simulink model "AE426SIMULINK8_OLD_viewerV2"  (R2024b)
settings: Solver=ode4  StartTime=0  StopTime=simlength  FixedStep=dt  RelTol=1e-3
InitFcn:
  | clear
  | clf
  | close all
  | wrlFilePath = fullfile(pwd, 'SpacecraftEarth.wrl');
  | myworld = vrworld(wrlFilePath);
  | open(myworld);
  | set(0,'Units','pixels');
  | 
  | screenSize = get(0, 'ScreenSize');
  | screenWidth = screenSize(3);
  | screenHeight = screenSize(4);
  | figWidth = screenWidth / 3;
  | figHeight = screenHeight / 2;
  | 
  | positions = [
  |      screenHeight - figHeight, 0, figWidth, figHeight; % Top-left
  |      figWidth, screenHeight - figHeight, figWidth, figHeight; % Top-right
  |      2*figWidth, screenHeight - figHeight, figWidth, figHeight; % Bottom-left
  | ];
  | 
  | fig1 = vrfigure(myworld,positions(1, :));
  | set(fig1,'Viewpoint','WorldView');
  | 
  | fig2 = vrfigure(myworld,positions(2, :));
  | set(fig2,'Viewpoint','NadirView');
  | 
  | fig3 = vrfigure(myworld,positions(3, :));
  | set(fig3,'Viewpoint','TargetView');
  | 
  | vrsetpref DefaultFigurePlaneClipMethod bvolume
  | 
  | % CONFIGURATION GOEMETRY MODELLING
  | 
  | fuse_dia = 0.3; % m
  | fuse_L = 0.9; %m
  | braket_space = 0.05; % m
  | num_ab = 3;
  | ab_span = 0.9; % m
  | ab_chord = 0.6844; % m
  | sys_CG = [-.01641,.06324,-.40481]; % m; respect to top of fuselage
  | 
  | CYLc = [0,0,.45] + sys_CG;
  | ab_cd = 2.2;
  | cyl_cd = 0.8;
  | 
  | mu = 3.986004e5;
  | dt = 0.01;
  | % ypr0 = [pi/4,pi/6,-pi/6];
  | % q1 = sin(ypr0(3)/2)*cos(ypr0(2)/2)*cos(ypr0(1)/2)-cos(ypr0(3)/2)*sin(ypr0(2)/2)*sin(ypr0(1)/2);
  | % q2 = sin(ypr0(3)/2)*cos(ypr0(2)/2)*sin(ypr0(1)/2)+cos(ypr0(3)/2)*sin(ypr0(2)/2)*cos(ypr0(1)/2);
  | % q3 = cos(ypr0(3)/2)*cos(ypr0(2)/2)*sin(ypr0(1)/2)-sin(ypr0(3)/2)*sin(ypr0(2)/2)*cos(ypr0(1)/2);
  | % q4 = cos(ypr0(3)/2)*cos(ypr0(2)/2)*cos(ypr0(1)/2)+sin(ypr0(3)/2)*sin(ypr0(2)/2)*sin(ypr0(1)/2);
  | % q0 = [q1;q2;q3;q4];
  | q0 = [0;0;0;1];
  | w0 = [0.000;0.000;0.000];
  | H0 = [0;0;0];
  | lat = [34.6178 34.9438 34.3658].*pi./180;
  | long = [-112.4503 -111.7529 -111.4481].*pi./180;
  | longlat = [long;lat]';
  | 
  | ... (+72 lines)
StopFcn:
  | data = get(out,"YPR");
  | data_e1 = get(out,"TargetYPR");
  | t = data.time - 51744.4;
  | 
  | y = data.Data(:,1);
  | p = data.Data(:,2);
  | r = data.Data(:,3);
  | ye = data_e1.Data(:,1);
  | pe = data_e1.Data(:,2);
  | re = data_e1.Data(:,3);
  | figure(1);
  | 
  | subplot(1,3,1);
  | hold on
  | plot(t, y*180/pi, 'b')
  | plot(t, ye*180/pi, '--r')
  | hold off
  | ylabel('Yaw (deg)')
  | xlabel('Time (s)')
  | grid on
  | 
  | subplot(1,3,2);
  | hold on
  | plot(t, p*180/pi, 'b')
  | plot(t, pe*180/pi, '--r')
  | hold off
  | ylabel('Pitch (deg)')
  | xlabel('Time (s)')
  | grid on
  | 
  | subplot(1,3,3);
  | hold on
  | plot(t, r*180/pi, 'b')
  | plot(t, re*180/pi, '--r')
  | hold off
  | ylabel('Roll (deg)')
  | xlabel('Time (s)')
  | grid on
  | 
  | data2 = get(out,"Torque");
  | t = data2.time - 51744.4;
  | 
  | y = data2.Data(3,:);
  | p = data2.Data(2,:);
  | r = data2.Data(1,:);
  | figure(2);
  | subplot(1,3,1);
  | plot(t, y, 'b')
  | ylabel('T_Y (N*m)')
  | xlabel('Time (s)')
  | grid on
  | subplot(1,3,2);
  | plot(t, p, 'b')
  | ylabel('T_P (N*m)')
  | xlabel('Time (s)')
  | grid on
  | subplot(1,3,3);
  | plot(t, r, 'b')
  | ylabel('T_R (N*m)')
  | xlabel('Time (s)')
  | ... (+23 lines)
undefined symbols (not defined in the file): K
libraries: matrix_library x16, vrlib x8, simulink x1, aerolibatmos2 x1
(part 2 of 2)

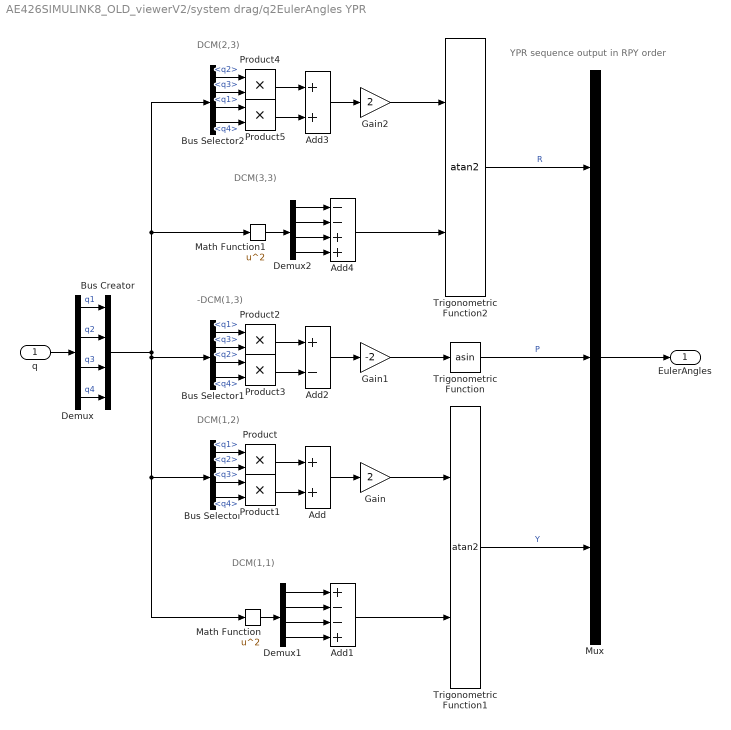
== system AE426SIMULINK8_OLD_viewerV2/system drag/q2EulerAngles YPR ==
  note: YPR sequence output in RPY order
  note: DCM(3,3)
  note: DCM(2,3)
  note: -DCM(1,3)
  note: DCM(1,1)
  note: DCM(1,2)
  q : Inport
  Add : Sum
  Add1 : Sum  Inputs=+--+
  Add2 : Sum  Inputs=+-
  Add3 : Sum
  Add4 : Sum  Inputs=--++
  Bus Creator : BusCreator  Inputs=4
  Bus Selector : BusSelector  OutputSignals=q1,q2,q3,q4
  Bus Selector1 : BusSelector  OutputSignals=q1,q3,q2,q4
  Bus Selector2 : BusSelector  OutputSignals=q2,q3,q1,q4
  Demux : Demux
  Demux1 : Demux
  Demux2 : Demux
  Gain : Gain  Gain=2
  Gain1 : Gain  Gain=-2
  Gain2 : Gain  Gain=2
  Math Function : Math  Operator=square
  Math Function1 : Math  Operator=square
  Mux : Mux  Inputs=3
  Product{,1..5} (6 alike) : Product
  Trigonometric Function : Trigonometry  Operator=asin
  Trigonometric Function1 : Trigonometry  Operator=atan2
  Trigonometric Function2 : Trigonometry  Operator=atan2
  EulerAngles : Outport  VectorParamsAs1DForOutWhenUnconnected=off
  wires:
  Add4/1 -> Trigonometric Function2/2
  Add1/1 -> Trigonometric Function1/2
  Gain/1 -> Trigonometric Function1/1
  Gain2/1 -> Trigonometric Function2/1
  Trigonometric Function2/1 -> Mux/1  "R"
  Trigonometric Function/1 -> Mux/2  "P"
  Trigonometric Function1/1 -> Mux/3  "Y"
  q/1 -> Demux/1
  Demux/1 -> Bus Creator/1  "q1"
  Demux/2 -> Bus Creator/2  "q2"
  Demux/3 -> Bus Creator/3  "q3"
  Demux/4 -> Bus Creator/4  "q4"
  Gain1/1 -> Trigonometric Function/1
  Bus Selector/3 -> Product1/1  "<q3>"
  Bus Selector/2 -> Product/2  "<q2>"
  Product1/1 -> Add/2
  Add/1 -> Gain/1
  Bus Selector/1 -> Product/1  "<q1>"
  Bus Selector/4 -> Product1/2  "<q4>"
  Product/1 -> Add/1
  Demux1/1 -> Add1/1
  Demux1/4 -> Add1/4
  Demux1/2 -> Add1/2
  Demux1/3 -> Add1/3
  Math Function/1 -> Demux1/1
  Bus Selector1/3 -> Product3/1  "<q2>"
  Product2/1 -> Add2/1
  Bus Selector1/4 -> Product3/2  "<q4>"
  Bus Selector1/1 -> Product2/1  "<q1>"
  Bus Selector1/2 -> Product2/2  "<q3>"
  Add2/1 -> Gain1/1
  Product3/1 -> Add2/2
  Bus Selector2/4 -> Product5/2  "<q4>"
  Bus Selector2/3 -> Product5/1  "<q1>"
  Bus Selector2/2 -> Product4/2  "<q3>"
  Bus Selector2/1 -> Product4/1  "<q2>"
  Product4/1 -> Add3/1
  Add3/1 -> Gain2/1
  Product5/1 -> Add3/2
  Demux2/1 -> Add4/1
  Demux2/4 -> Add4/4
  Demux2/2 -> Add4/2
  Demux2/3 -> Add4/3
  Math Function1/1 -> Demux2/1
  Bus Creator/1 -> Math Function/1, Bus Selector/1, Bus Selector1/1, Bus Selector2/1, Math Function1/1
  Mux/1 -> EulerAngles/1

== system AE426SIMULINK8_OLD_viewerV2/system drag/r to rho ==
  r : Inport
  Cast To Double : DataTypeConversion  OutDataTypeStr=double  SaturateOnIntegerOverflow=off  RndMeth=Floor
  Constant : Constant  Value=Rn
  Dot Product : DotProduct  OutDataTypeStr=Inherit: Inherit via internal rule
  ISA Atmosphere Model : aerolibatmos2/ISA Atmosphere Model  useExtended=on  action=Warning  custom=off  viscosityOut=off  g=9.80665  gamma=1.4  R=287.0531  L=0.0065  h_trop=11000  h_strat=20000  rho0=1.225  P0=101325  T0=288.15  h0=0  S=110.4  Tref=273.15  muref=1.716e-5
  Scope : Scope
  Sqrt : Sqrt
  Subtract : Sum  Inputs=+-
  rho : Outport
  wires:
  Dot Product/1 -> Sqrt/1
  Subtract/1 -> Cast To Double/1
  Sqrt/1 -> Subtract/1
  Constant/1 -> Subtract/2
  r/1 -> Dot Product/2, Dot Product/1
  Cast To Double/1 -> ISA Atmosphere Model/1
  ISA Atmosphere Model/4 -> Scope/1, rho/1

== system AE426SIMULINK8_OLD_viewerV2/Animation/Nadir EOM/q2EulerParameters ==
  qNF : Inport
  Demux : Demux  Outputs=[3,1]
  Divide1 : Product  Inputs=*/
  Gain1 : Gain  Gain=2
  Mux : Mux  Inputs=2
  Trigonometric Function : Trigonometry  Operator=acos
  Trigonometric Function1 : Trigonometry
  "e, phi" : Outport
  wires:
  Mux/1 -> "e, phi"/1  "e, phi"
  Gain1/1 -> Mux/2  "phi"
  Demux/1 -> Divide1/1  "qhat"
  Demux/2 -> Trigonometric Function/1  "q4"
  Trigonometric Function1/1 -> Divide1/2  "phi/2"
  Trigonometric Function/1 -> Gain1/1, Trigonometric Function1/1  "phi/2"
  Divide1/1 -> Mux/1  "e"
  qNF/1 -> Demux/1

== system AE426SIMULINK8_OLD_viewerV2/Animation/qOrbit wrt Inertial/DCM2q ==
  DCM : Inport
  Bus Creator : BusCreator  Inputs=9
  Bus Selector : BusSelector  OutputSignals=DCM(11),DCM(22),DCM(33),DCM(23),DCM(32),DCM(31),DCM(13),DCM(12),DCM(21)
  Constant : Constant
  Demux : Demux  Outputs=9
  Divide : Product  Inputs=/*
  Gain : Gain  Gain=0.5
  Gain1 : Gain  Gain=4
  Mux : Mux  Inputs=2
  Mux1 : Mux  Inputs=3
  Square Root : Sqrt
  Sum : Sum  Inputs=++++
  Sum1 : Sum  Inputs=+-
  Sum2 : Sum  Inputs=+-
  Sum3 : Sum  Inputs=+-
  q : Outport
  wires:
  Divide/1 -> Mux/1
  Gain1/1 -> Divide/1
  Mux1/1 -> Divide/2
  Sum3/1 -> Mux1/3
  Sum2/1 -> Mux1/2
  Sum1/1 -> Mux1/1
  Bus Selector/9 -> Sum3/2  "<DCM(21)>"
  Bus Selector/8 -> Sum3/1  "<DCM(12)>"
  Bus Selector/7 -> Sum2/2  "<DCM(13)>"
  Bus Selector/6 -> Sum2/1  "<DCM(31)>"
  Mux/1 -> q/1
  Gain/1 -> Gain1/1, Mux/2
  Bus Selector/5 -> Sum1/2  "<DCM(32)>"
  Bus Selector/4 -> Sum1/1  "<DCM(23)>"
  Square Root/1 -> Gain/1
  Sum/1 -> Square Root/1
  Constant/1 -> Sum/4
  Bus Selector/3 -> Sum/3  "<DCM(33)>"
  Bus Selector/2 -> Sum/2  "<DCM(22)>"
  Bus Selector/1 -> Sum/1  "<DCM(11)>"
  Bus Creator/1 -> Bus Selector/1
  Demux/9 -> Bus Creator/9  "DCM(33)"
  Demux/8 -> Bus Creator/8  "DCM(32)"
  Demux/7 -> Bus Creator/7  "DCM(31)"
  Demux/6 -> Bus Creator/6  "DCM(23)"
  Demux/5 -> Bus Creator/5  "DCM(22)"
  Demux/4 -> Bus Creator/4  "DCM(21)"
  Demux/3 -> Bus Creator/3  "DCM(13)"
  Demux/2 -> Bus Creator/2  "DCM(12)"
  Demux/1 -> Bus Creator/1  "DCM(11)"
  DCM/1 -> Demux/1

== system AE426SIMULINK8_OLD_viewerV2/Vehicle Dynamics/Quaternion & Omega EOMs/first term of w dot BO ==
  I^-1 : Inport
  T : Inport  Port=2
  I : Inport  Port=3
  omega B/F : Inport  Port=4
  Add : Sum
  Constant : Constant  Value=H0
  Cross Product : matrix_library/Cross Product
  Matrix Multiply1 : Product  Multiplication=Matrix(*)
  MatrixMultiply1 : Product  Multiplication=Matrix(*)
  Sum : Sum  Inputs=+-
  first term : Outport
  wires:
  Cross Product/1 -> Sum/2
  Constant/1 -> Add/2
  omega B/F/1 -> Matrix Multiply1/2, Cross Product/1
  I^-1/1 -> MatrixMultiply1/1
  I/1 -> Matrix Multiply1/1
  Matrix Multiply1/1 -> Add/1
  Add/1 -> Cross Product/2
  Sum/1 -> MatrixMultiply1/2
  T/1 -> Sum/1
  MatrixMultiply1/1 -> first term/1

== system AE426SIMULINK8_OLD_viewerV2/Vehicle Dynamics/Quaternion & Omega EOMs/omega OF dot EOM ==
  qDCM_BO : Inport
  w_BO : Inport  Port=2
  -theta_double_dot : Inport  Port=3
  -theta_dot : Inport  Port=4
  Add : Sum
  Demux1 : Demux  Outputs=3
  Gain5 : Gain  Gain=[0 0 0; 0 0 1; 0 -1 0]
  Gain6 : Gain  Gain=[ 0 1 0; -1 0 0; 0 0 0]
  Gain7 : Gain  Gain=[0 0 -1; 0 0 0; 1 0 0]
  Matrix Multiply : Product  Multiplication=Matrix(*)
  Matrix Multiply2 : Product  Multiplication=Matrix(*)
  Matrix Multiply3 : Product  Multiplication=Matrix(*)
  Sum3 : Sum  Inputs=+++
  w dot OF : Outport
  omega O/F : Outport  Port=2
  wires:
  qDCM_BO/1 -> Matrix Multiply2/1, Matrix Multiply/1
  Demux1/1 -> Gain5/1
  Demux1/2 -> Gain7/1
  Gain5/1 -> Sum3/1
  Matrix Multiply/1 -> omega O/F/1, Matrix Multiply3/2  "omega O/F"
  Sum3/1 -> Matrix Multiply3/1
  Gain7/1 -> Sum3/2
  Demux1/3 -> Gain6/1
  Gain6/1 -> Sum3/3
  -theta_double_dot/1 -> Matrix Multiply2/2  "-theta double dot"
  -theta_dot/1 -> Matrix Multiply/2  "-theta_dot"
  Matrix Multiply2/1 -> Add/2  "omerga dot O/F part1"
  w_BO/1 -> Demux1/1  "w_BO"
  Matrix Multiply3/1 -> Add/1  "omega dot OF part 2"
  Add/1 -> w dot OF/1

== system AE426SIMULINK8_OLD_viewerV2/Vehicle Dynamics/Quaternion & Omega EOMs/q EOM ==
  note: $\dot\bar q = \frac 1 2 \Omega \bar q$
  q : Inport
  w : Inport  Port=2
  Demux : Demux  Outputs=3
  Gain : Gain  Gain=[0 0 0 1; 0 0 1 0; 0 -1 0 0; -1 0 0 0]
  Gain1 : Gain  Gain=[0 0 -1 0; 0 0 0 1; 1 0 0 0; 0 -1 0 0]
  Gain2 : Gain  Gain=[0 1 0 0; -1 0 0 0; 0 0 0 1; 0 0 -1 0]
  Gain3 : Gain  Gain=0.5
  MatrixMultiply : Product  Multiplication=Matrix(*)
  Sum : Sum  Inputs=+++
  q_dot : Outport
  wires:
  w/1 -> Demux/1
  Demux/2 -> Gain1/1
  Demux/1 -> Gain/1
  Demux/3 -> Gain2/1
  Gain1/1 -> Sum/2
  Gain2/1 -> Sum/3
  Gain/1 -> Sum/1
  Sum/1 -> Gain3/1
  MatrixMultiply/1 -> q_dot/1  "q_dot"
  Gain3/1 -> MatrixMultiply/1
  q/1 -> MatrixMultiply/2

== system AE426SIMULINK8_OLD_viewerV2/Vehicle Dynamics/Quaternion & Omega EOMs/q2DCM ==
  q : Inport
  Add : Sum  Inputs=-+
  Add1 : Sum  Inputs=+++
  Add2 : Sum  Inputs=+++
  Demux : Demux  Outputs=3
  Demux2 : Demux  Outputs=[3,1]
  Divide : Product  Inputs=**
  Gain : Gain  Gain=2
  Gain2 : Gain  Gain=[0 0 0;0 0 2;0 -2 0]
  Gain3 : Gain  Gain=[0 0 -2;0 0 0;2 0 0]
  Gain4 : Gain  Gain=[0 2 0;-2 0 0;0 0 0]
  Gain5 : Gain  Gain=eye(3)
  Math Function : Math  Operator=square
  Matrix Multiply : Product  Multiplication=Matrix(*)
  Matrix Multiply1 : Product  Multiplication=Matrix(*)
  Transpose : matrix_library/Transpose
  DCM : Outport
  wires:
  Math Function/1 -> Add/2
  Matrix Multiply1/1 -> Add/1
  Add2/1 -> Divide/2
  Gain/1 -> Add1/1
  Transpose/1 -> Matrix Multiply1/1, Matrix Multiply/2
  Demux/2 -> Gain3/1  "q2"
  Gain3/1 -> Add2/2
  Demux2/2 -> Divide/1, Math Function/1  "q4"
  Matrix Multiply/1 -> Gain/1
  Demux/1 -> Gain2/1  "q1"
  Gain5/1 -> Add1/2
  Divide/1 -> Add1/3
  Gain2/1 -> Add2/1
  Demux/3 -> Gain4/1  "q3"
  Gain4/1 -> Add2/3
  Add/1 -> Gain5/1
  Demux2/1 -> Matrix Multiply1/2, Transpose/1, Matrix Multiply/1, Demux/1  "qhat"
  q/1 -> Demux2/1
  Add1/1 -> DCM/1

== system AE426SIMULINK8_OLD_viewerV2/Vehicle Dynamics/Quaternion & Omega EOMs/thetas ==
  r : Inport
  v : Inport  Port=2
  Cross Product1 : matrix_library/Cross Product
  Divide : Product  Inputs=/*
  Divide1 : Product  Inputs=*/*
  Dot Product : DotProduct  OutDataTypeStr=Inherit: Inherit via internal rule
  Dot Product1 : DotProduct  OutDataTypeStr=Inherit: Inherit via internal rule
  Dot Product2 : DotProduct  OutDataTypeStr=Inherit: Inherit via internal rule
  Gain3 : Gain  Gain=[0;-1;0]
  Gain4 : Gain  Gain=-2
  Sqrt : Sqrt
  -theta double dot : Outport
  -theta dot : Outport  Port=2
  wires:
  Divide/1 -> Gain3/1  "theta dot"
  Dot Product/1 -> Sqrt/1
  v/1 -> Cross Product1/2, Dot Product2/1
  Dot Product1/1 -> Divide1/2, Divide/1  "r^2"
  Gain3/1 -> -theta dot/1, Divide1/3  "-theta dot"
  Divide1/1 -> Gain4/1
  Cross Product1/1 -> Dot Product/1, Dot Product/2
  r/1 -> Cross Product1/1, Dot Product1/1, Dot Product1/2, Dot Product2/2
  Sqrt/1 -> Divide/2
  Dot Product2/1 -> Divide1/1
  Gain4/1 -> -theta double dot/1  "-theta double dot"

== system AE426SIMULINK8_OLD_viewerV2/system drag/Aibrake Coords/AC_ab1 ==
  In1 : Inport
  Constant : Constant  Value=fuse_dia/2+braket_space
  Constant1 : Constant  Value=0
  Constant2 : Constant  Value=ab_span/2
  Constant3 : Constant  Value=ab_span/2
  Cos : Trigonometry  Operator=cos
  Mux : Mux  Inputs=3
  Product : Product
  Product1 : Product
  Reshape : Reshape  OutputDimensionality=Row vector (2-D)
  Sin : Trigonometry
  Sum : Sum  Inputs=|++
  Outport : Outport
  wires:
  Reshape/1 -> Outport/1
  Sum/1 -> Mux/1
  Product1/1 -> Mux/3
  Constant3/1 -> Product/2
  Product/1 -> Sum/1
  Constant2/1 -> Product1/1
  Sin/1 -> Product/1
  Constant1/1 -> Mux/2
  In1/1 -> Sin/1, Cos/1
  Constant/1 -> Sum/2
  Mux/1 -> Reshape/1
  Cos/1 -> Product1/2

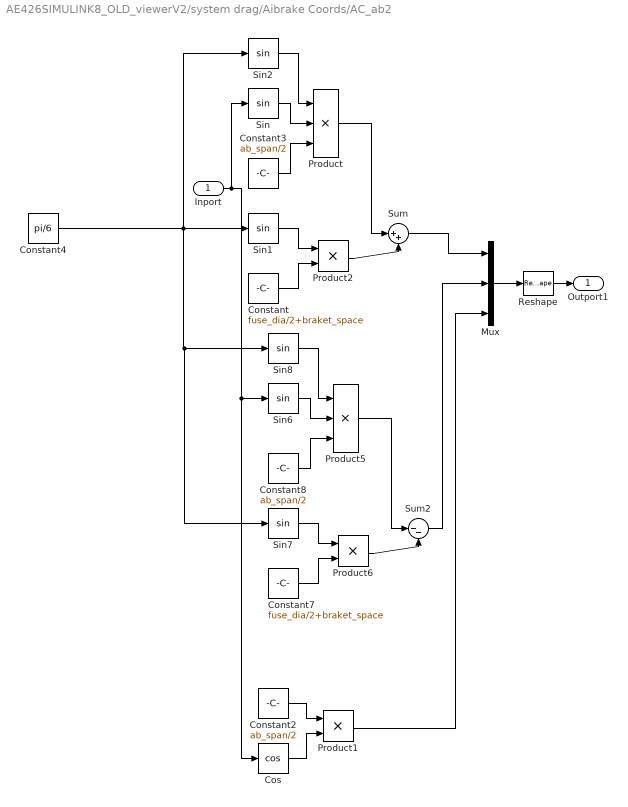
== system AE426SIMULINK8_OLD_viewerV2/system drag/Aibrake Coords/AC_ab2 ==
  Inport : Inport
  Constant : Constant  Value=fuse_dia/2+braket_space
  Constant2 : Constant  Value=ab_span/2
  Constant3 : Constant  Value=ab_span/2
  Constant4 : Constant  Value=pi/6
  Constant7 : Constant  Value=fuse_dia/2+braket_space
  Constant8 : Constant  Value=ab_span/2
  Cos : Trigonometry  Operator=cos
  Mux : Mux  Inputs=3
  Product : Product  Inputs=3
  Product1 : Product
  Product2 : Product
  Product5 : Product  Inputs=3
  Product6 : Product
  Reshape : Reshape  OutputDimensionality=Row vector (2-D)
  Sin{,1..2,6..8} (6 alike) : Trigonometry
  Sum : Sum  Inputs=|++
  Sum2 : Sum  Inputs=|--
  Outport1 : Outport
  wires:
  Sum2/1 -> Mux/2
  Constant7/1 -> Product6/2
  Product6/1 -> Sum2/2
  Product5/1 -> Sum2/1
  Sin8/1 -> Product5/1
  Sin7/1 -> Product6/1
  Constant8/1 -> Product5/3
  Sin6/1 -> Product5/2
  Constant4/1 -> Sin1/1, Sin2/1, Sin8/1, Sin7/1
  Sin2/1 -> Product/1
  Sin/1 -> Product/2
  Constant3/1 -> Product/3
  Product2/1 -> Sum/2
  Constant/1 -> Product2/2
  Sin1/1 -> Product2/1
  Reshape/1 -> Outport1/1
  Sum/1 -> Mux/1
  Product1/1 -> Mux/3
  Product/1 -> Sum/1
  Constant2/1 -> Product1/1
  Inport/1 -> Sin/1, Cos/1, Sin6/1
  Mux/1 -> Reshape/1
  Cos/1 -> Product1/2

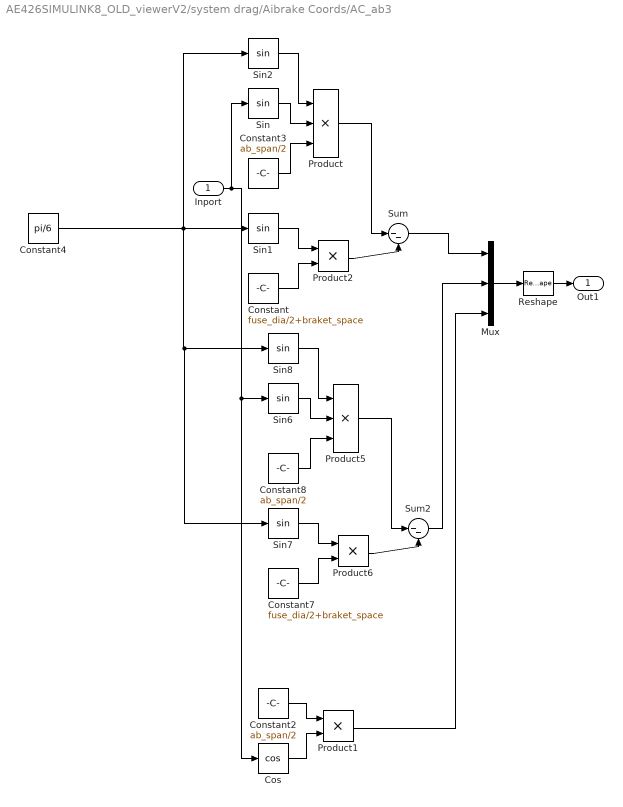
== system AE426SIMULINK8_OLD_viewerV2/system drag/Aibrake Coords/AC_ab3 ==
  Inport : Inport
  Constant : Constant  Value=fuse_dia/2+braket_space
  Constant2 : Constant  Value=ab_span/2
  Constant3 : Constant  Value=ab_span/2
  Constant4 : Constant  Value=pi/6
  Constant7 : Constant  Value=fuse_dia/2+braket_space
  Constant8 : Constant  Value=ab_span/2
  Cos : Trigonometry  Operator=cos
  Mux : Mux  Inputs=3
  Product : Product  Inputs=3
  Product1 : Product
  Product2 : Product
  Product5 : Product  Inputs=3
  Product6 : Product
  Reshape : Reshape  OutputDimensionality=Row vector (2-D)
  Sin{,1..2,6..8} (6 alike) : Trigonometry
  Sum : Sum  Inputs=|--
  Sum2 : Sum  Inputs=|--
  Out1 : Outport
  wires:
  Sum2/1 -> Mux/2
  Constant7/1 -> Product6/2
  Product6/1 -> Sum2/2
  Product5/1 -> Sum2/1
  Sin8/1 -> Product5/1
  Sin7/1 -> Product6/1
  Constant8/1 -> Product5/3
  Sin6/1 -> Product5/2
  Constant4/1 -> Sin1/1, Sin2/1, Sin8/1, Sin7/1
  Sin2/1 -> Product/1
  Sin/1 -> Product/2
  Constant3/1 -> Product/3
  Product2/1 -> Sum/2
  Constant/1 -> Product2/2
  Sin1/1 -> Product2/1
  Reshape/1 -> Out1/1
  Sum/1 -> Mux/1
  Product1/1 -> Mux/3
  Product/1 -> Sum/1
  Constant2/1 -> Product1/1
  Inport/1 -> Sin/1, Cos/1, Sin6/1
  Mux/1 -> Reshape/1
  Cos/1 -> Product1/2

== system AE426SIMULINK8_OLD_viewerV2/system drag/Airbrake system lift/Airbrake Lift1 ==
  Velocity : Inport
  rho : Inport  Port=2
  delta : Inport  Port=3
  Position : Inport  Port=4
  Constant : Constant  Value=0.5
  Constant2 : Constant  Value=0
  Cross Product : matrix_library/Cross Product
  Demux : Demux  Outputs=3
  Divide : Product  Inputs=*/
  Dot Product : DotProduct  OutDataTypeStr=Inherit: Inherit via internal rule
  Mux : Mux  Inputs=3
  Product : Product  Inputs=7
  Span*Chord : Constant  Value=ab_span*ab_chord
  Sqrt : Sqrt
  cL_delta : Constant  Value=ab_cd
  ab_Lift : Outport
  wires:
  Span*Chord/1 -> Product/7
  Constant/1 -> Product/6
  rho/1 -> Product/5
  delta/1 -> Product/2
  cL_delta/1 -> Product/1
  Product/1 -> ab_Lift/1
  Cross Product/1 -> Product/4, Product/3
  Dot Product/1 -> Sqrt/1
  Sqrt/1 -> Divide/2
  Position/1 -> Demux/1
  Demux/2 -> Mux/2
  Demux/1 -> Mux/1
  Constant2/1 -> Mux/3
  Mux/1 -> Cross Product/2
  Divide/1 -> Cross Product/1
  Velocity/1 -> Dot Product/2, Dot Product/1, Divide/1

== system AE426SIMULINK8_OLD_viewerV2/system drag/Airbrake system lift/Airbrake Lift2 ==
  Velocity : Inport
  rho : Inport  Port=2
  delta : Inport  Port=3
  In1 : Inport  Port=4
  Constant : Constant  Value=0.5
  Constant1 : Constant  Value=ab_span*ab_chord
  Constant2 : Constant  Value=0
  Cross Product : matrix_library/Cross Product
  Demux : Demux  Outputs=3
  Divide : Product  Inputs=*/
  Dot Product : DotProduct  OutDataTypeStr=Inherit: Inherit via internal rule
  Mux : Mux  Inputs=3
  Product : Product  Inputs=7
  Sqrt : Sqrt
  cL_delta : Constant  Value=ab_cd
  ab_Lift : Outport
  wires:
  Divide/1 -> Cross Product/1
  Mux/1 -> Cross Product/2
  Constant2/1 -> Mux/3
  Demux/1 -> Mux/1
  Demux/2 -> Mux/2
  In1/1 -> Demux/1
  Sqrt/1 -> Divide/2
  Cross Product/1 -> Product/3, Product/4
  Product/1 -> ab_Lift/1
  cL_delta/1 -> Product/1
  delta/1 -> Product/2
  rho/1 -> Product/5
  Constant/1 -> Product/6
  Constant1/1 -> Product/7
  Dot Product/1 -> Sqrt/1
  Velocity/1 -> Dot Product/2, Dot Product/1, Divide/1

== system AE426SIMULINK8_OLD_viewerV2/system drag/Airbrake system lift/Airbrake Lift3 ==
  Velocity : Inport
  rho : Inport  Port=2
  delta : Inport  Port=3
  In1 : Inport  Port=4
  Constant : Constant  Value=0.5
  Constant1 : Constant  Value=ab_span*ab_chord
  Constant2 : Constant  Value=0
  Cross Product : matrix_library/Cross Product
  Demux : Demux  Outputs=3
  Divide : Product  Inputs=*/
  Dot Product : DotProduct  OutDataTypeStr=Inherit: Inherit via internal rule
  Mux : Mux  Inputs=3
  Product : Product  Inputs=7
  Sqrt : Sqrt
  cL_delta : Constant  Value=ab_cd
  ab_Lift : Outport
  wires:
  Constant1/1 -> Product/7
  Constant/1 -> Product/6
  rho/1 -> Product/5
  cL_delta/1 -> Product/1
  Product/1 -> ab_Lift/1
  Cross Product/1 -> Product/4, Product/3
  Sqrt/1 -> Divide/2
  In1/1 -> Demux/1
  Demux/2 -> Mux/2
  Demux/1 -> Mux/1
  Constant2/1 -> Mux/3
  Mux/1 -> Cross Product/2
  Divide/1 -> Cross Product/1
  delta/1 -> Product/2
  Dot Product/1 -> Sqrt/1
  Velocity/1 -> Dot Product/2, Dot Product/1, Divide/1
